simulink model "state_looper_model"  (R2015b)
settings: Solver=VariableStepAuto  StartTime=0.0  StopTime=inf  RelTol=1e-3
settings Model: Creator=tech  LastModifiedBy=tech

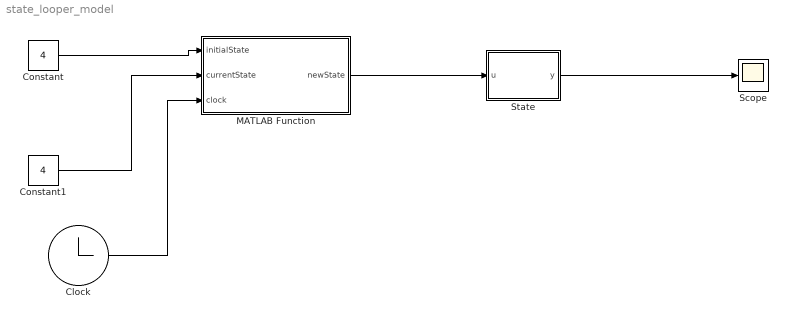
== system state_looper_model ==
  Clock : Clock
  Constant : Constant  Value=4
  Constant1 : Constant  Value=4
  MATLAB Function : MATLAB Function  TreatAsAtomicUnit=on
  Scope : Scope
  State : MATLAB Function  TreatAsAtomicUnit=on
  wires:
  State/1(y) -> Scope/1
  Constant/1 -> MATLAB Function/1(initialState)
  MATLAB Function/1(newState) -> State/1(u)
  Constant1/1 -> MATLAB Function/2(currentState)
  Clock/1 -> MATLAB Function/3(clock)

== matlab function state_looper_model/MATLAB Function ==
  data: initialState input; newState output; currentState input; clock input
function newState = fcn(initialState, currentState, clock)

states = [1 2 4 8];
newState = 8;

if(initialState ~= 8 && clock > 2)
    pause(0.1);
    for i = 1 : length(states)
        if(states(i) == currentState && i < 4)
            newState = states(i+1);
        end
    end
else
    newState = initialState;
end

== matlab function state_looper_model/State ==
  data: u input; y output
function y = fcn(u)
%#codegen

y = u;
